simulink model "model_4"  (R2021b)
settings: Solver=FixedStepAuto  StartTime=0.0  StopTime=15  FixedStep=0.001  RelTol=1e-3
values from neighbouring files (symbols this model uses):
  A1 = [10, 7, 8; 2, 15, 10; 3, 11, 12]    [task_1.m]    (also in task_3.m = [1, 1, 0; -1, 1, 0; 0, 0, -3]; task_4.m = [1, 1, 0; -1, 1, 0; 0, 0, -3]; task_5.m = [0 1; 0 0]; untitled2.m = [-3 0 0; 0 4 2; 0 -2 4])
  A2 = [0.5, 2, 0, 0; -2, 0.5, 0, 0; 0, 0, 0.3, 1; 0, 0, -1, 0.3]    [task_1.m]    (also in task_3.m = [0 5 0; -5 0 0; 0 0 0.01]; task_4.m = [0 5 0; -5 0 0; 0 0 0.01]; task_5.m = [0 1 0 0 0 0; -1 0 0 0 0 0; 0 0 0 3 0 0; 0 0 -3 0 0 0; untitled2.m = [0 5 0 0; -5 0 0 0; 0 0 0 2; 0 0 -2 0])
  B1 = [1;2;3]    [task_1.m]    (also in task_3.m = [1;1;1]; task_4.m = [1;1;1]; task_5.m = [0; 1]; untitled2.m = [1; 1; 1])
  B2 = [1, 1, 1, 1; 1, 2, 3, 4; 1, 2, 3, 4]    [task_1.m]    (also in task_3.m = [1,1,1;1,1,1;1,1,1]; task_4.m = [1,1,1;1,1,1;1,1,1]; task_5.m = [0 0 0 0 0 0; 0 0 0 0 0 0]; untitled2.m = [1 0 0 0; 0 1 0 0; 0 0 1 1])
  C1 = [1,0,1]    [task_3.m]    (also in task_4.m = [1,1,1]; task_5.m = [1 0]; untitled2.m = [1 0 1])
  C2 = [1, 1, 1]    [task_1.m]    (also in task_3.m; task_4.m; task_5.m = -C1; untitled2.m = [1 1 1])
  D1 = [1,1,0]    [task_3.m]    (also in task_4.m = [-1,-1,-1]; task_5.m = [1 0 1 0 1 0]; untitled2.m = [1 1 0 0])
  D2 = zeros(1, 4)    [task_1.m]    (also in task_3.m = [-1, -1, -1]; task_4.m = [-1, -1, -1]; task_5.m = [8/pi 0 8/(3*pi) 0 8/(5*pi) 0]; untitled2.m = [-1 -1 -1 -1])
  K1 = -Y1*inv(P1)    [task_1.m]    (also in task_3.m; task_4.m; task_5.m = -y*inv(p); untitled2.m = -y*inv(p))
  K2 = Y2 - K1*P2    [task_1.m]    (also in task_3.m; task_4.m; task_5.m = Y - K1*P; untitled2.m = Y - K1*P)
  L1 = l(1:3)    [task_3.m]    (also in task_4.m; task_5.m = l(1:2); untitled2.m)
  L2 = l(4:6)    [task_3.m]    (also in task_4.m; task_5.m = l(3:8); untitled2.m = l(4:7))
settings Model: Creator=den  LastModifiedBy=vital

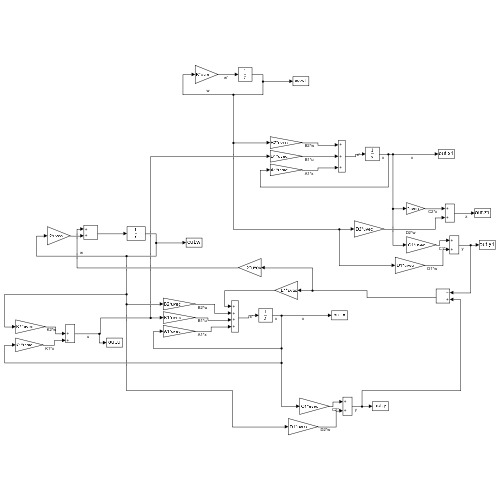
[thumbnail: Simulink's stored preview of the top-level diagram]
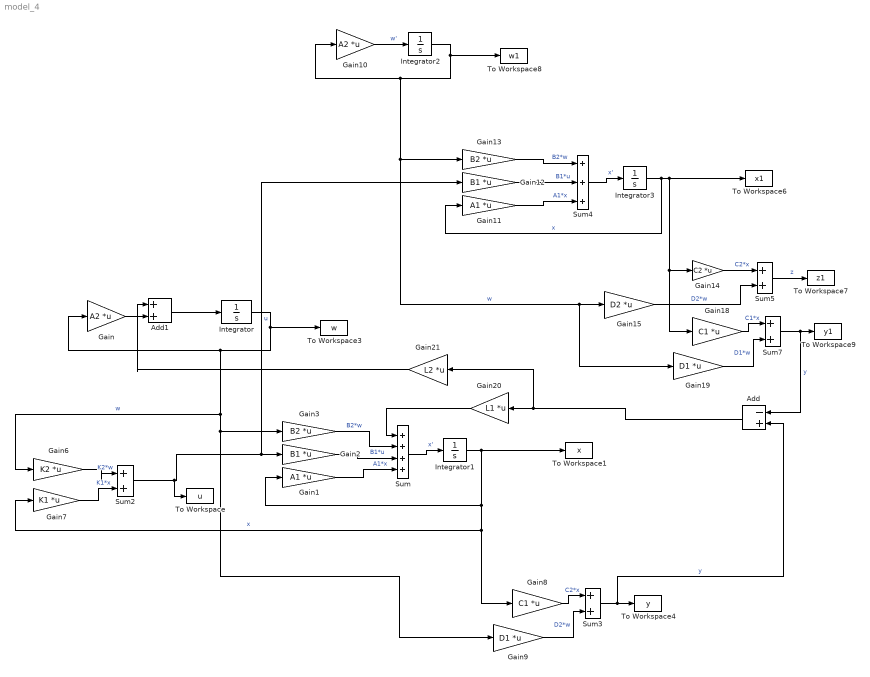
== system model_4 ==
  Add : Sum  Inputs=-+
  Add1 : Sum
  Gain : Gain  Gain=A2  Multiplication=Matrix(K*u) (u vector)
  Gain1 : Gain  Gain=A1  Multiplication=Matrix(K*u) (u vector)
  Gain10 : Gain  Gain=A2  Multiplication=Matrix(K*u) (u vector)
  Gain11 : Gain  Gain=A1  Multiplication=Matrix(K*u) (u vector)
  Gain12 : Gain  Gain=B1  Multiplication=Matrix(K*u) (u vector)
  Gain13 : Gain  Gain=B2  Multiplication=Matrix(K*u) (u vector)
  Gain14 : Gain  Gain=C2  Multiplication=Matrix(K*u) (u vector)
  Gain15 : Gain  Gain=D2  Multiplication=Matrix(K*u) (u vector)
  Gain18 : Gain  Gain=C1  Multiplication=Matrix(K*u) (u vector)
  Gain19 : Gain  Gain=D1  Multiplication=Matrix(K*u) (u vector)
  Gain2 : Gain  Gain=B1  Multiplication=Matrix(K*u) (u vector)
  Gain20 : Gain  Gain=L1  Multiplication=Matrix(K*u) (u vector)
  Gain21 : Gain  Gain=L2  Multiplication=Matrix(K*u) (u vector)
  Gain3 : Gain  Gain=B2  Multiplication=Matrix(K*u) (u vector)
  Gain6 : Gain  Gain=K2  Multiplication=Matrix(K*u) (u vector)
  Gain7 : Gain  Gain=K1  Multiplication=Matrix(K*u) (u vector)
  Gain8 : Gain  Gain=C1  Multiplication=Matrix(K*u) (u vector)
  Gain9 : Gain  Gain=D1  Multiplication=Matrix(K*u) (u vector)
  Integrator : Integrator  InitialCondition=[0;0;0]
  Integrator1 : Integrator  InitialCondition=[0;0;0]
  Integrator2 : Integrator  InitialCondition=[1;1;1]
  Integrator3 : Integrator  InitialCondition=[0;0;0]
  Sum : Sum  Inputs=++++
  Sum2 : Sum  Inputs=|++
  Sum3 : Sum
  Sum4 : Sum  Inputs=+++
  Sum5 : Sum
  Sum7 : Sum
  To Workspace : ToWorkspace  VariableName=u  SaveFormat=Timeseries  SampleTime=-1
  To Workspace1 : ToWorkspace  VariableName=x  SaveFormat=Timeseries  SampleTime=-1
  To Workspace3 : ToWorkspace  VariableName=w  SaveFormat=Timeseries  SampleTime=-1
  To Workspace4 : ToWorkspace  VariableName=y  SaveFormat=Timeseries  SampleTime=-1
  To Workspace6 : ToWorkspace  VariableName=x1  SaveFormat=Timeseries  SampleTime=0.001
  To Workspace7 : ToWorkspace  VariableName=z1  SaveFormat=Timeseries  SampleTime=-1
  To Workspace8 : ToWorkspace  VariableName=w1  SaveFormat=Timeseries  SampleTime=-1
  To Workspace9 : ToWorkspace  VariableName=y1  SaveFormat=Timeseries  SampleTime=-1
  wires:
  Integrator/1 -> To Workspace3/1, Gain6/1, Gain9/1, Gain3/1, Gain/1  "w"
  Sum/1 -> Integrator1/1  "x'"
  Integrator1/1 -> To Workspace1/1, Gain7/1, Gain8/1, Gain1/1  "x"
  Gain7/1 -> Sum2/2  "K1*x"
  Sum2/1 -> To Workspace/1, Gain12/1, Gain2/1  "u"
  Gain6/1 -> Sum2/1  "K2*w"
  Gain1/1 -> Sum/4  "A1*x"
  Gain2/1 -> Sum/3  "B1*u"
  Gain3/1 -> Sum/2  "B2*w"
  Gain9/1 -> Sum3/2  "D2*w"
  Gain8/1 -> Sum3/1  "C2*x"
  Sum3/1 -> Add/2, To Workspace4/1  "y"
  Gain19/1 -> Sum7/2  "D1*w"
  Sum7/1 -> Add/1, To Workspace9/1  "y"
  Integrator2/1 -> To Workspace8/1, Gain19/1, Gain15/1, Gain13/1, Gain10/1  "w"
  Gain18/1 -> Sum7/1  "C1*x"
  Gain15/1 -> Sum5/2  "D2*w"
  Integrator3/1 -> To Workspace6/1, Gain18/1, Gain14/1, Gain11/1  "x"
  Gain14/1 -> Sum5/1  "C2*x"
  Sum4/1 -> Integrator3/1  "x'"
  Gain10/1 -> Integrator2/1  "w'"
  Sum5/1 -> To Workspace7/1  "z"
  Gain11/1 -> Sum4/3  "A1*x"
  Gain12/1 -> Sum4/2  "B1*u"
  Gain13/1 -> Sum4/1  "B2*w"
  Add/1 -> Gain21/1, Gain20/1
  Gain20/1 -> Sum/1
  Gain/1 -> Add1/2
  Add1/1 -> Integrator/1
  Gain21/1 -> Add1/1
